simulink model "communicationTesting"  (R2020a)
settings: Solver=FixedStepAuto  StartTime=0.0  StopTime=inf  FixedStep=.005  RelTol=1e-3
libraries: xpcrtudplib x2, dspnetwork x2, simulink x1, ptplib x1, etargetslib x1, xpcutilitieslib x1
settings Model: xpc_rtwmakecfg_data=_xpcnblib__xpcetherlib__xpcether8255xlib__xpcetherGbElib__xpciplib_  Creator=Hiwi  LastModifiedBy=Hiwi

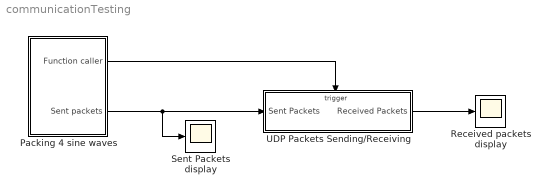
== system communicationTesting ==
  Packing 4 sine waves : Subsystem
  Received packets display : Scope
  Sent Packets display : Scope
  UDP Packets Sending/Receiving : Subsystem  TreatAsAtomicUnit=on
  wires:
  UDP Packets Sending/Receiving/1(Received Packets) -> Received packets display/1
  Packing 4 sine waves/1(Function caller) -> UDP Packets Sending/Receiving/Trigger
  Packing 4 sine waves/2(Sent packets) -> Sent Packets display/1, UDP Packets Sending/Receiving/1(Sent Packets)

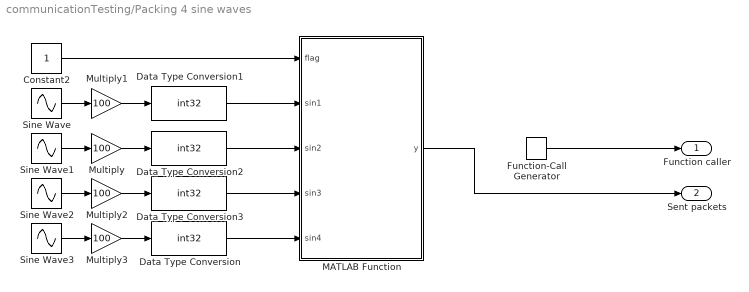
== system communicationTesting/Packing 4 sine waves ==
  Constant2 : Constant  OutDataTypeStr=int32
  Data Type Conversion{,1..3} (4 alike) : DataTypeConversion  OutDataTypeStr=int32
  Function-Call Generator : simulink/Ports & Subsystems/Function-Call Generator  sample_time=1  numberOfIterations=1
  MATLAB Function : MATLAB Function  TreatAsAtomicUnit=on
  Multiply{,1..3} (4 alike) : Gain  Gain=100
  Sine Wave : Sin  SampleTime=0
  Sine Wave1 : Sin  Phase=pi/4  SampleTime=0
  Sine Wave2 : Sin  Phase=pi/2  SampleTime=0
  Sine Wave3 : Sin  Frequency=.5  Phase=pi  SampleTime=0
  Function caller : Outport
  Sent packets : Outport  Port=2
  wires:
  Sine Wave2/1 -> Multiply2/1
  Data Type Conversion2/1 -> MATLAB Function/3(sin2)
  Multiply2/1 -> Data Type Conversion3/1
  Sine Wave3/1 -> Multiply3/1
  Sine Wave1/1 -> Multiply/1
  Multiply3/1 -> Data Type Conversion/1
  Sine Wave/1 -> Multiply1/1
  Multiply1/1 -> Data Type Conversion1/1
  Multiply/1 -> Data Type Conversion2/1
  Data Type Conversion/1 -> MATLAB Function/5(sin4)
  Data Type Conversion3/1 -> MATLAB Function/4(sin3)
  Data Type Conversion1/1 -> MATLAB Function/2(sin1)
  Constant2/1 -> MATLAB Function/1(flag)
  Function-Call Generator/1 -> Function caller/1
  MATLAB Function/1(y) -> Sent packets/1

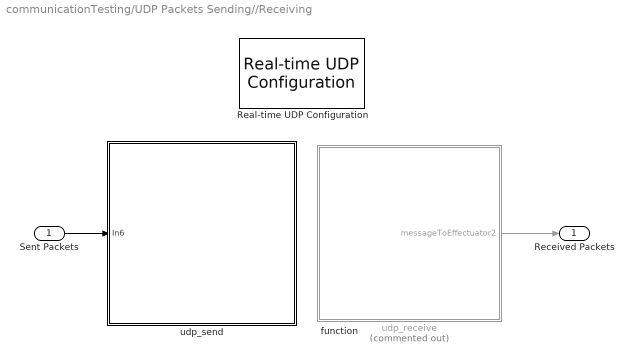
== system communicationTesting/UDP Packets Sending//Receiving ==
  Sent Packets : Inport
  function : TriggerPort  TriggerType=function-call  VariantControl=Variant
  "Real-time UDP Configuration " : ptplib/PTP UDP/Real-time UDP  Configuration   ID=1  IpAddress=192.168.5.90  SubnetMask=255.255.255.0  Gateway=0.0.0.0  EthDrv=Intel Gigabit  PciBus=5  PciSlot=0  PciFunction=0  udpID=0  MulticastList=[]  Multicast={}
      settings: SourceProductBaseCode=XP
  udp_receive : Subsystem  Commented=on
  udp_send : Subsystem
  Received Packets : Outport
  wires:
  Sent Packets/1 -> udp_send/1(In6)
  udp_receive/1(messageToEffectuator2) -> Received Packets/1

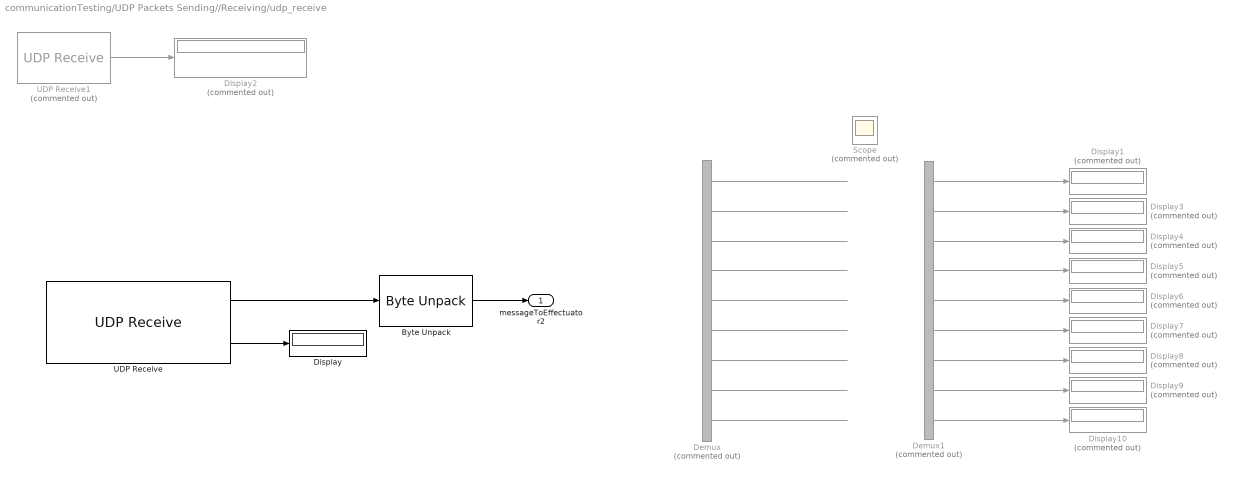
== system communicationTesting/UDP Packets Sending//Receiving/udp_receive ==
  Byte Unpack : etargetslib/Byte Unpack  dimensions={[9]}  datatypes={'int32'}  byteAlign=1
  Demux : Demux  Commented=on  Outputs=9
  Demux1 : Demux  Commented=on  Outputs=9
  Display : Display
  Display{1..10} (10 alike) : Display  Commented=on
  Scope : Scope  Commented=on
  UDP Receive : xpcrtudplib/UDP Receive  ipAddressVal=Use host-target connection  localPort=8000  rcvWidth=9*4  rcvFmAny=off  fmAddress=192.168.5.100  rcvMulticast=off  multicastAddress={}  maxUDPQueue=8  sampleTime=-1
  UDP Receive1 : dspnetwork/UDP Receive  Commented=on  localURL='0.0.0.0'  localPort=8000  remoteURL='192.168.5.100'  remotePort=-1  recvBufferSize=8192  dims=255  signalDatatype=uint32  isComplex=off  isVarSize=on  showBlockingTime=on  blockingTime=inf  sampletime=0.01  blockPlatform=HOST
  messageToEffectuator2 : Outport
  wires:
  UDP Receive/2 -> Display/1
  UDP Receive/1 -> Byte Unpack/1
  Demux/4 -> ?
  Demux/3 -> ?
  Demux/2 -> ?
  Demux/1 -> ?
  UDP Receive1/1 -> Display2/1
  Demux/5 -> ?
  Demux/6 -> ?
  Demux/7 -> ?
  Demux/8 -> ?
  Demux1/8 -> Display9/1
  Demux1/7 -> Display8/1
  Demux1/6 -> Display7/1
  Demux1/5 -> Display6/1
  Demux1/1 -> Display1/1
  Demux1/2 -> Display3/1
  Demux1/3 -> Display4/1
  Demux1/4 -> Display5/1
  Demux/9 -> ?
  Demux1/9 -> Display10/1
  Byte Unpack/1 -> messageToEffectuator2/1

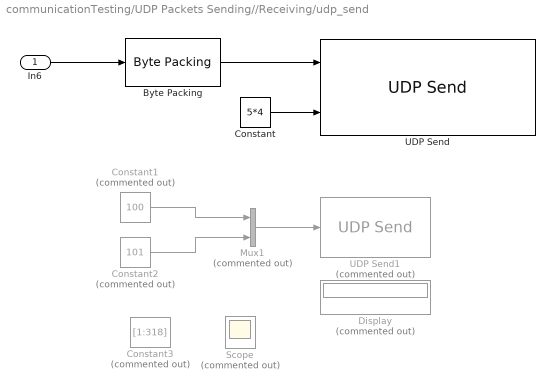
== system communicationTesting/UDP Packets Sending//Receiving/udp_send ==
  In6 : Inport
  "Byte Packing " : xpcutilitieslib/Byte Packing   MaskPackedDataType=uint8  MaskUnpackedDataTypes={'int32'}  MaskAlignment=1
  Constant : Constant  Value=5*4
  Constant1 : Constant  Commented=on  Value=100
  Constant2 : Constant  Commented=on  Value=101
  Constant3 : Constant  Commented=on  Value=[1:318]  OutDataTypeStr=int32
  Display : Display  Commented=on
  Mux1 : Mux  Commented=on  Inputs=2
  Scope : Scope  Commented=on
  UDP Send : xpcrtudplib/UDP Send  ipAddressVal=Use host-target connection  localPort=8080  toAddress=192.168.5.100  toPort=8080  sampleTime=-1
      settings: SourceProductBaseCode=XP
  UDP Send1 : dspnetwork/UDP Send  Commented=on  remoteURL='192.168.5.100'  remotePort=10  localURL='0.0.0.0'  localPortSource=Specify via dialog  localPort=8000  sendBufferSize=8192  sampletime=-1  blockPlatform=HOST  separateLengthPort=0
  wires:
  Constant/1 -> UDP Send/2
  "Byte Packing "/1 -> UDP Send/1
  Mux1/1 -> UDP Send1/1
  Constant1/1 -> Mux1/1
  Constant2/1 -> Mux1/2
  In6/1 -> "Byte Packing "/1

== matlab function communicationTesting/Packing 4 sine waves/MATLAB Function ==
  data: flag input; y output; sin1 input; sin2 input; sin3 input; sin4 input
function y = fcn(flag,sin1,sin2,sin3,sin4)

y = [flag;sin1;sin2;sin3;sin4];
